simulink subsystem "SchlittenGleichungKraft"  (R2020a)
settings: Solver=VariableStepAuto  StartTime=0.0  StopTime=10.0  RelTol=1e-3
settings Model: Creator=Tobias  LastModifiedBy=Tobias

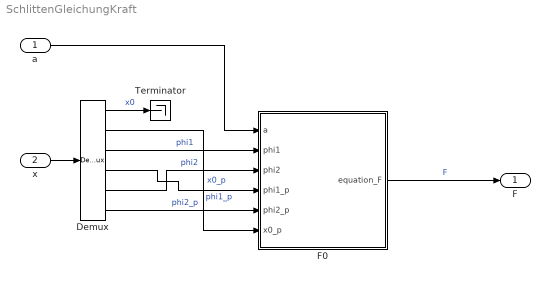
== system SchlittenGleichungKraft ==
  a : Inport
  x : Inport  Port=2
  Demux : Demux  Outputs=6
  F0 : MATLAB Function  TreatAsAtomicUnit=on
  Terminator : Terminator
  F : Outport
  wires:
  Demux/5 -> F0/3(phi2)  "phi2"
  F0/1(equation_F) -> F/1  "F"
  a/1 -> F0/1(a)
  Demux/1 -> Terminator/1  "x0"
  Demux/2 -> F0/6(x0_p)  "x0_p"
  Demux/4 -> F0/4(phi1_p)  "phi1_p"
  x/1 -> Demux/1
  Demux/6 -> F0/5(phi2_p)  "phi2_p"
  Demux/3 -> F0/2(phi1)  "phi1"

== matlab function SchlittenGleichungKraft/F0 ==
  data: a input; equation_F output; phi1 input; phi2 input; phi1_p input; phi2_p input; x0_p input
function equation_F = F0(a,phi1,phi2,phi1_p,phi2_p,x0_p)
%#codegen

%    This function was generated by the Symbolic Math Toolbox version 8.5.
%    02-Sep-2020 15:58:01

t2 = cos(phi1);
t3 = cos(phi2);
t4 = phi1.*2.0;
t5 = phi2.*2.0;
t6 = phi1_p.^2;
t7 = phi2_p.^2;
t10 = -phi2;
t12 = x0_p.*1.0e+2;
t8 = cos(t4);
t9 = cos(t5);
t11 = -t5;
t13 = tanh(t12);
t16 = t4+t10;
t14 = phi1+t11;
t17 = t4+t11;
t18 = cos(t16);
t20 = t9.*9.45065076121045e-6;
t21 = t8.*1.420522013890127e-4;
t15 = cos(t14);
t19 = cos(t17);
t22 = -t20;
t23 = t19.*3.671558484319389e-3;
t24 = t21+t22+t23-1.177154833778282e-2;
equation_F = (t24.*(a-(t13.*1.116853755464231e-2+x0_p.*1.169696515703051e-2-sin(t4).*1.393532095626215e-3+sin(t5).*9.271088396747451e-5+phi1_p.*t2.*2.603497104619667e-5-phi1_p.*t3.*1.251140377267428e-6-phi2_p.*t2.*1.836182779980471e-6+phi2_p.*t3.*1.251140377267428e-6-phi1_p.*t15.*7.299879136949721e-6+phi2_p.*t15.*5.14842607023521e-7+phi1_p.*t18.*1.508756513646403e-6-phi2_p.*t18.*1.508756513646403e-6-t13.*t19.*3.515838913523943e-3-t19.*x0_p.*3.682187132202257e-3+t6.*sin(phi1).*7.27408278246111e-5+t7.*sin(phi2).*9.803464946644989e-6+t6.*sin(t14).*2.745414046131636e-6+t7.*sin(t16).*1.408151648240494e-5)./t24))./(t19.*2.16599243070721e-4-6.88056773942971e-4);
